simulink model "PIEstimator"  (Simulink 10.0)
settings: Solver=ode3  StartTime=0.0  StopTime=Tsim  FixedStep=deltat  RelTol=1e-3  EnableMultiTasking=on
values from neighbouring files (symbols this model uses):
  a = 0    [Q4.m]    (also in Sol_Q1.m = 0.1)
  alpha2 = 3*a    (= 0.3)    [Sol_Q1.m]
  dAmp = 20    [Sol_Q1.m]    (also in main3.m = -3; param3.m = -2)
  delay = 0.5    [Sol_Q1.m]    (also in main3.m = 0; param3.m = 0.01; params2.m = 5)
  deltat = 0.01    [Q4.m]    (also in Sol_Q1.m = 0.001; main3.m; param3.m = 0.001; params2.m = 0.1)
  Gs = tf(b, [1 a])    [Q4.m]    (also in Q5.m = tf([b1 b0], [1 a1 a0]); Sol_Q1.m = tf(num, den); main3.m = tf(num, den); param3.m = tf(b, [1 a1 a0]))
  K1 = (alpha1 - a)/b    (= 1.5)    [Q4.m]    (also in Sol_Q1.m = 5; main3.m = 4; param3.m = 5)
  K2 = alpha2/b    (= 15)    [Sol_Q1.m]    (also in main3.m = 2.121; param3.m = 2.121)
  Tsim = 20    [Sol_Q1.m]    (also in main3.m = 10)
  umax = 8.8    [Q4.m]    (also in Sol_Q1.m = 10000; main3.m = 4.5; param3.m = 999)
  umin = -100    [Q4.m]    (also in Sol_Q1.m = -10000; main3.m = -0.9; param3.m = -999)
settings Model: Creator=e50128  LastModifiedBy=adityaaaap
settings DataIOCC: LimitDataPoints=on  SignalLoggingSaveFormat=ModelDataLogs
settings OptimizationCC: ExpressionDepthLimit=2147483647
settings DebuggingCC: SolverPrmCheckMsg=warning  FcnCallInpInsideContextMsg=warning  StateNameClashWarn=warning
settings GRTTargetCC: GeneratePreprocessorConditionals=Disable all
settings ConfigComp: CovExternalEMLEnable=off

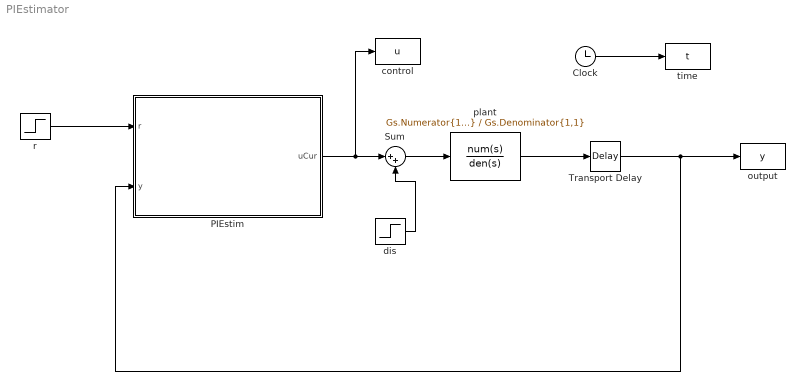
== system PIEstimator ==
  Clock : Clock
  PIEstim : MATLAB Function  TreatAsAtomicUnit=on
  Sum : Sum  Inputs=|++
  Transport Delay : TransportDelay  DelayTime=delay
  control : ToWorkspace  VariableName=u
      settings: MaxDataPoints=100000
  dis : Step  Time=Tsim/2  After=dAmp  SampleTime=0
  output : ToWorkspace  VariableName=y
      settings: MaxDataPoints=100000
  plant : TransferFcn  Numerator=Gs.Numerator{1,1}  Denominator=Gs.Denominator{1,1}
  r : Step  Time=0  SampleTime=0
  time : ToWorkspace  VariableName=t
      settings: MaxDataPoints=100000
  wires:
  r/1 -> PIEstim/1(r)
  Clock/1 -> time/1
  plant/1 -> Transport Delay/1
  Transport Delay/1 -> output/1, PIEstim/2(y)
  PIEstim/1(uCur) -> Sum/1, control/1
  dis/1 -> Sum/2
  Sum/1 -> plant/1

== matlab function PIEstim ==
  settings: updateMethod=DISCRETE  sampleTime=deltat
  data: uCur output double; r input double; y input double; K1 parameter double; K2 parameter double; alpha2 parameter double; a parameter double; deltat parameter double; umin parameter double; umax parameter double
function uCur = PIEstim(r,y,K1,K2,alpha2,a,deltat,umin,umax)
persistent zhat
if isempty(zhat)
    zhat=0;
end
%estimator based MATLAB function with anti-windup
dhat=zhat+K2*(y-r);
uCur= -K1*(y-r)-dhat; 
if (uCur>umax) uCur=umax;end
if (uCur<umin) uCur=umin;end
%zhat=zhat-alpha2*zhat*deltat-deltat*(y-r)*K2*(alpha2-a)-deltat*alpha2*udelay(1,ndmax);
zhat=zhat-alpha2*zhat*deltat-deltat*(y-r)*K2*(alpha2-a)-deltat*alpha2*uCur;
